simulink subsystem "MAG"  (R2025b)
settings: Solver=VariableStepAuto  StartTime=0.0  StopTime=10.0  RelTol=1e-3
model mask{magUpdateFreq=1, magMeasLim=0, magNoisePerChannel=0, magNoiseSeed=0}
  mask prompts: magUpdateFreq "Update frequency [Hz]"; magMeasLim "Measurement range [nT]"; magNoisePerChannel "Noise per channel (3 sigma) [nT]"; magNoiseSeed "Noise seeds"
settings Model: Creator=antoniohernandez-rodiciomateos  LastModifiedBy=antoniohernandez-rodiciomateos

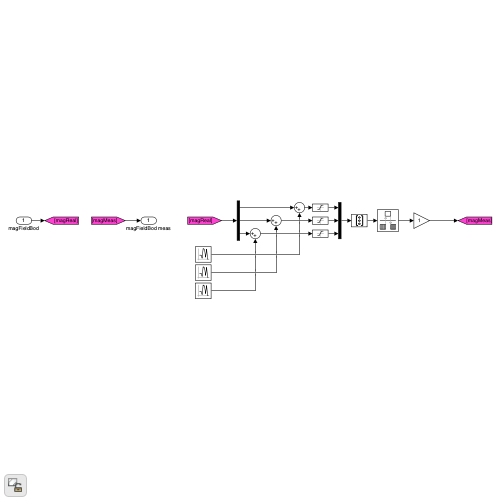
[thumbnail: Simulink's stored preview of the top-level diagram]
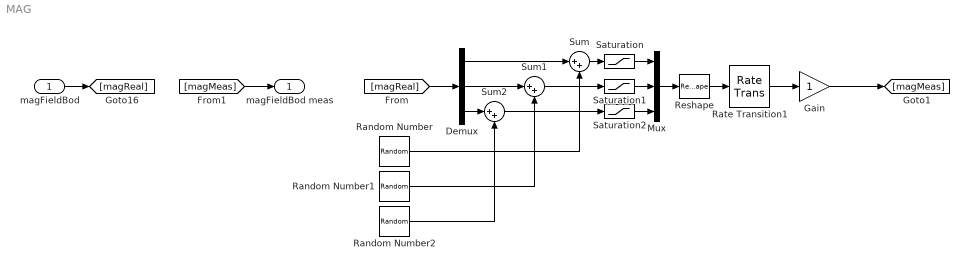
== system MAG ==
  magFieldBod : Inport  PortDimensions=[3 1]
  Demux : Demux  Outputs=3
  Gain : Gain
  Mux : Mux  Inputs=3
  Random Number : RandomNumber  Variance=(magNoisePerChannel ^ 2) / 9  Seed=magNoiseSeed(1)  SampleTime=1 / magUpdateFreq
  Random Number1 : RandomNumber  Variance=(magNoisePerChannel ^ 2) / 9  Seed=magNoiseSeed(2)  SampleTime=1 / magUpdateFreq
  Random Number2 : RandomNumber  Variance=(magNoisePerChannel ^ 2) / 9  Seed=magNoiseSeed(3)  SampleTime=1 / magUpdateFreq
  Rate Transition1 : RateTransition  OutPortSampleTime=1 / magUpdateFreq
  Reshape : Reshape  OutputDimensionality=Column vector (2-D)
  Saturation : Saturate  UpperLimit=magMeasLim  LowerLimit=-1 * magMeasLim
  Saturation1 : Saturate  UpperLimit=magMeasLim  LowerLimit=-1 * magMeasLim
  Saturation2 : Saturate  UpperLimit=magMeasLim  LowerLimit=-1 * magMeasLim
  Sum : Sum  Inputs=|++
  Sum1 : Sum  Inputs=|++
  Sum2 : Sum  Inputs=|++
  magFieldBod meas : Outport  PortDimensions=[3 1]
  wires:
  [magReal] -> Demux/1
  Demux/1 -> Sum/1
  Random Number/1 -> Sum/2
  Demux/2 -> Sum1/1
  Demux/3 -> Sum2/1
  Random Number1/1 -> Sum1/2
  Random Number2/1 -> Sum2/2
  [magMeas] -> magFieldBod meas/1
  Mux/1 -> Reshape/1
  Saturation/1 -> Mux/1
  Sum/1 -> Saturation/1
  Saturation1/1 -> Mux/2
  Sum1/1 -> Saturation1/1
  Saturation2/1 -> Mux/3
  Sum2/1 -> Saturation2/1
  magFieldBod/1 -> [magReal]
  Reshape/1 -> Rate Transition1/1
  Gain/1 -> [magMeas]
  Rate Transition1/1 -> Gain/1
